simulink model "IPMSM_SVC"  (R2023a)
settings: Solver=FixedStepDiscrete  StartTime=0.0  StopTime=10.0  RelTol=1e-3
model workspace (MATLAB code in the model file):
  | cmdLim = Simulink.Parameter;
  | cmdLim.Value = 15;
  | cmdLim.Description = 'Limit for controlling the maximum surface command angle.';
  | cmdLim.Min = 0;
  | cmdLim.Max = 90;
  | cmdLim.DocUnits = 'deg';
  | 
  | dispGain = Simulink.Parameter;
  | dispGain.Value = 0.75;
  | dispGain.Description = 'Gain applied to the displacement error.';
  | dispGain.Min = 0;
  | dispGain.Max = [];
  | dispGain.DocUnits = 'deg/sec/deg';
  | 
  | dispLim = Simulink.Parameter;
  | dispLim.Value = 30;
  | dispLim.Description = 'Limit for controlling the maximum commanded angle.';
  | dispLim.Min = 0;
  | dispLim.Max = 180;
  | dispLim.DocUnits = 'deg';
  | 
  | intGain = Simulink.Parameter;
  | intGain.Value = 0.5;
  | intGain.Description = 'Gain applied to the integral error.';
  | intGain.Min = 0;
  | intGain.Max = [];
  | intGain.DocUnits = 'deg/sec/deg/sec';
  | 
  | intLim = Simulink.Parameter;
  | intLim.Value = 5;
  | intLim.Description = 'Limit for controlling the maximum commanded angle.';
  | intLim.Min = 0;
  | intLim.Max = 90;
  | intLim.DocUnits = 'deg';
  | 
  | rateGain = Simulink.Parameter;
  | rateGain.Value = 2;
  | rateGain.Description = 'Gain applied to the rate error.';
  | rateGain.Min = 0;
  | rateGain.Max = [];
  | rateGain.DocUnits = 'deg/deg/sec';
  | 
  | rateLim = Simulink.Parameter;
  | rateLim.Value = 6;
  | rateLim.Description = 'Limit for controlling the maximum commanded angle.';
  | rateLim.Min = 0;
  | rateLim.Max = 180;
  | rateLim.DocUnits = 'deg/sec';
  | 
  | hdgGain = Simulink.Parameter;
  | hdgGain.Value = 0.015;
settings Model: RequirementInfo={} %GIDa_fe9045fd_0412_4b6e_8206_617cc20e6fde  Creator=洲  LastModifiedBy=洲
settings SolverCC: AlgebraicLoopSolver=TrustRegion  AutoInsertRateTranBlk=on
settings DataIOCC: SaveOutput=off  SignalLogging=off  DSMLogging=off  SaveTime=off
settings OptimizationCC: DefaultParameterBehavior=Inlined  UseDivisionForNetSlopeComputation=on  GainParamInheritBuiltInType=on  UseFloatMulNetSlope=on  UseSpecifiedMinMax=on  InlineInvariantSignals=on  EnhancedBackFolding=on  PassReuseOutputArgsAs=Individual arguments  ZeroExternalMemoryAtStartup=off  ZeroInternalMemoryAtStartup=off  NoFixptDivByZeroProtection=on  EfficientFloat2IntCast=on  LifeSpan=1  OptimizeBlockOrder=speed  DifferentSizesBufferReuse=on  OptimizationCustomize=off  EfficientTunableParamExpr=on
settings DebuggingCC: AllowSymbolicDim=off  SFUnexpectedBacktrackingDiag=warning  SFNoUnconditionalDefaultTransitionDiag=warning  SFExecutionAtInitializationDiag=none  ArithmeticOperatorsInVariantConditions=warning
settings HardwareCC: ProdLongLongMode=on
settings SFSimCC: MATLABDynamicMemAlloc=off
settings RTWCC: Description=Embedded Coder  SystemTargetFile=ert.tlc  TemplateMakefile=ert_default_tmf  BuildConfiguration=Faster Runs  DataTypeReplacement=CDataTypesFixedWidth
settings CodeAppCC: ForceParamTrailComments=on  IgnoreCustomStorageClasses=off  OperatorAnnotations=on  SimulinkDataObjDesc=on  SFDataObjDesc=on  CustomSymbolStrGlobalVar=rt$N$M  CustomSymbolStrType=$N$M  CustomSymbolStrFcn=$N$M$F  CustomSymbolStrMacro=$N$M  InsertBlockDesc=on  EnableCustomComments=on  ReqsInCode=on
settings ERTTargetCC: TargetLangStandard=C99 (ISO)  UtilityFuncGeneration=Shared location  MultiwordLength=2048  GenerateSampleERTMain=on  IncludeMdlTerminateFcn=off  CombineSignalStateStructs=on  SuppressErrorStatus=on  SupportAbsoluteTime=off  SupportNonFinite=off  SupportComplex=off  InlinedParameterPlacement=NonHierarchical  ERTCustomFileTemplate=example_file_process.tlc  ERTFilePackagingFormat=CompactWithDataFile
settings ConfigComp: CovScope=ReferencedModels  CovSaveName=covdata_rollAP  CovMetricSettings=dcmtrwe  CovHTMLOptions=-sRT=1 -aTS=1 -bRG=1 -bTC=1 -hTR=1 -nFC=0 -scm=1 -bcm=1 -xEv=0  CovSaveCumulativeToWorkspaceVar=on  CovSaveSingleToWorkspaceVar=on  CovCumulativeVarName=covCumulativeData_rollAP  CovReportOnPause=off  CovExternalEMLEnable=off  CovSFcnEnable=off

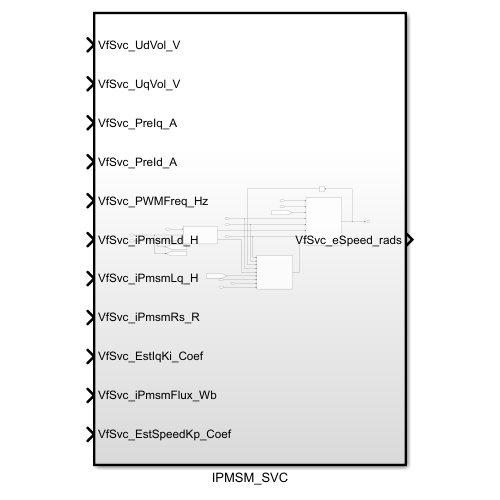
[thumbnail: Simulink's stored preview of the top-level diagram]
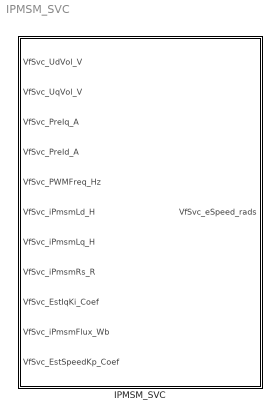
== system IPMSM_SVC ==
  IPMSM_SVC : Subsystem  TreatAsAtomicUnit=on
      settings: RTWSystemCode=Nonreusable function

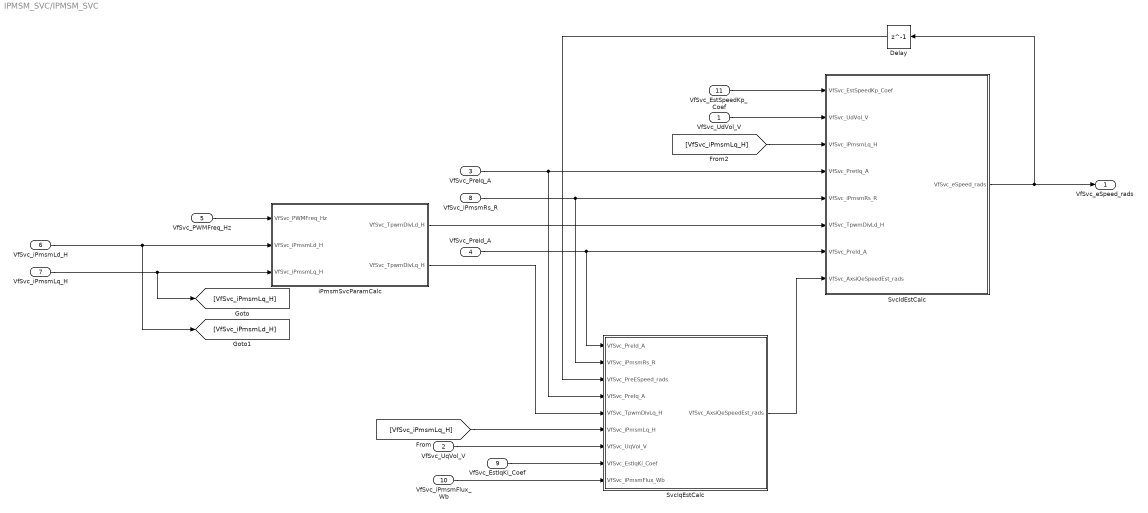
== system IPMSM_SVC/IPMSM_SVC ==
  VfSvc_UdVol_V : Inport
  VfSvc_UqVol_V : Inport  Port=2
  VfSvc_PreIq_A : Inport  Port=3
  VfSvc_PreId_A : Inport  Port=4
  VfSvc_PWMFreq_Hz : Inport  Port=5
  VfSvc_iPmsmLd_H : Inport  Port=6
  VfSvc_iPmsmLq_H : Inport  Port=7
  VfSvc_iPmsmRs_R : Inport  Port=8
  VfSvc_EstIqKi_Coef : Inport  Port=9
  VfSvc_iPmsmFlux_Wb : Inport  Port=10
  VfSvc_EstSpeedKp_Coef : Inport  Port=11
  Delay : Delay  DelayLength=1
  SvcIdEstCalc : Subsystem
  SvcIqEstCalc : Subsystem
  iPmsmSvcParamCalc : Subsystem  TreatAsAtomicUnit=on
      settings: RTWSystemCode=Nonreusable function  RTWFcnNameOpts=Use subsystem name
  VfSvc_eSpeed_rads : Outport
  wires:
  iPmsmSvcParamCalc/1(VfSvc_TpwmDivLd_H) -> SvcIdEstCalc/6(VfSvc_TpwmDivLd_H)
  SvcIqEstCalc/1(VfSvc_AxsiQeSpeedEst_rads) -> SvcIdEstCalc/8(VfSvc_AxsiQeSpeedEst_rads)
  VfSvc_iPmsmLq_H/1 -> iPmsmSvcParamCalc/3(VfSvc_iPmsmLq_H), [VfSvc_iPmsmLq_H]
  VfSvc_PreIq_A/1 -> SvcIqEstCalc/4(VfSvc_PreIq_A), SvcIdEstCalc/4(VfSvc_PretIq_A)
  VfSvc_iPmsmFlux_Wb/1 -> SvcIqEstCalc/9(VfSvc_iPmsmFlux_Wb)
  VfSvc_iPmsmRs_R/1 -> SvcIqEstCalc/2(VfSvc_iPmsmRs_R), SvcIdEstCalc/5(VfSvc_iPmsmRs_R)
  VfSvc_PWMFreq_Hz/1 -> iPmsmSvcParamCalc/1(VfSvc_PWMFreq_Hz)
  SvcIdEstCalc/1(VfSvc_eSpeed_rads) -> VfSvc_eSpeed_rads/1, Delay/1
  iPmsmSvcParamCalc/2(VfSvc_TpwmDivLq_H) -> SvcIqEstCalc/5(VfSvc_TpwmDivLq_H)
  VfSvc_PreId_A/1 -> SvcIqEstCalc/1(VfSvc_PreId_A), SvcIdEstCalc/7(VfSvc_PreId_A)
  VfSvc_iPmsmLd_H/1 -> [VfSvc_iPmsmLd_H], iPmsmSvcParamCalc/2(VfSvc_iPmsmLd_H)
  VfSvc_UdVol_V/1 -> SvcIdEstCalc/2(VfSvc_UdVol_V)
  VfSvc_UqVol_V/1 -> SvcIqEstCalc/7(VfSvc_UqVol_V)
  [VfSvc_iPmsmLq_H] -> SvcIqEstCalc/6(VfSvc_iPmsmLq_H)
  VfSvc_EstIqKi_Coef/1 -> SvcIqEstCalc/8(VfSvc_EstIqKi_Coef)
  VfSvc_EstSpeedKp_Coef/1 -> SvcIdEstCalc/1(VfSvc_EstSpeedKp_Coef)
  Delay/1 -> SvcIqEstCalc/3(VfSvc_PreESpeed_rads)
  [VfSvc_iPmsmLq_H] -> SvcIdEstCalc/3(VfSvc_iPmsmLq_H)

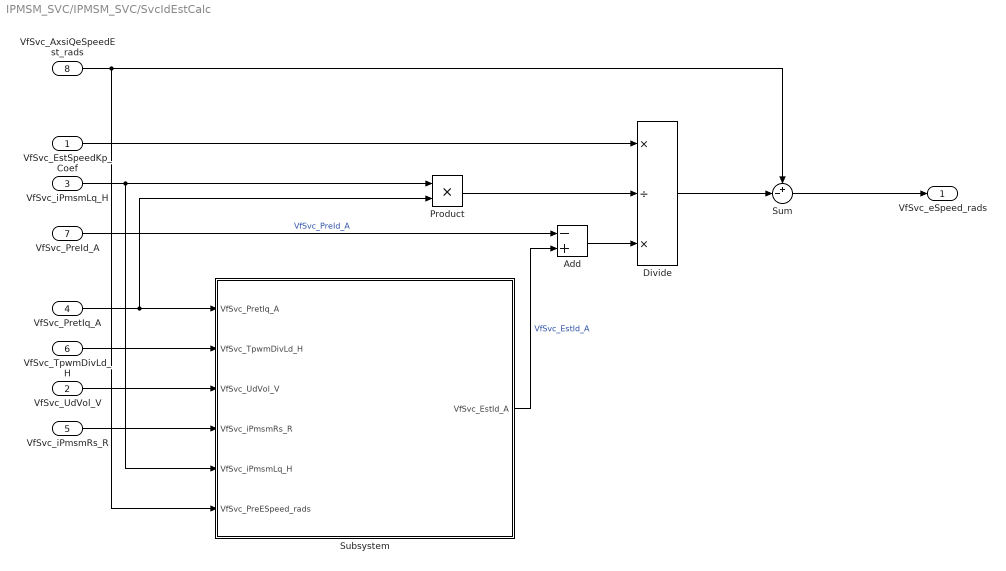
== system IPMSM_SVC/IPMSM_SVC/SvcIdEstCalc ==
  VfSvc_EstSpeedKp_Coef : Inport
  VfSvc_UdVol_V : Inport  Port=2
  VfSvc_iPmsmLq_H : Inport  Port=3
  VfSvc_PretIq_A : Inport  Port=4
  VfSvc_iPmsmRs_R : Inport  Port=5
  VfSvc_TpwmDivLd_H : Inport  Port=6
  VfSvc_PreId_A : Inport  Port=7
  VfSvc_AxsiQeSpeedEst_rads : Inport  Port=8
  Add : Sum  Inputs=-+
  Divide : Product  Inputs=*/*
  Product : Product
  Subsystem : Subsystem
  Sum : Sum  Inputs=+-|
  VfSvc_eSpeed_rads : Outport
  wires:
  VfSvc_TpwmDivLd_H/1 -> Subsystem/2(VfSvc_TpwmDivLd_H)
  VfSvc_UdVol_V/1 -> Subsystem/3(VfSvc_UdVol_V)
  VfSvc_PretIq_A/1 -> Product/2, Subsystem/1(VfSvc_PretIq_A)
  VfSvc_iPmsmRs_R/1 -> Subsystem/4(VfSvc_iPmsmRs_R)
  VfSvc_iPmsmLq_H/1 -> Subsystem/5(VfSvc_iPmsmLq_H), Product/1
  Subsystem/1(VfSvc_EstId_A) -> Add/2  "VfSvc_EstId_A"
  VfSvc_EstSpeedKp_Coef/1 -> Divide/1
  Add/1 -> Divide/3
  VfSvc_PreId_A/1 -> Add/1  "VfSvc_PreId_A"
  Divide/1 -> Sum/2
  VfSvc_AxsiQeSpeedEst_rads/1 -> Sum/1, Subsystem/6(VfSvc_PreESpeed_rads)
  Sum/1 -> VfSvc_eSpeed_rads/1
  Product/1 -> Divide/2

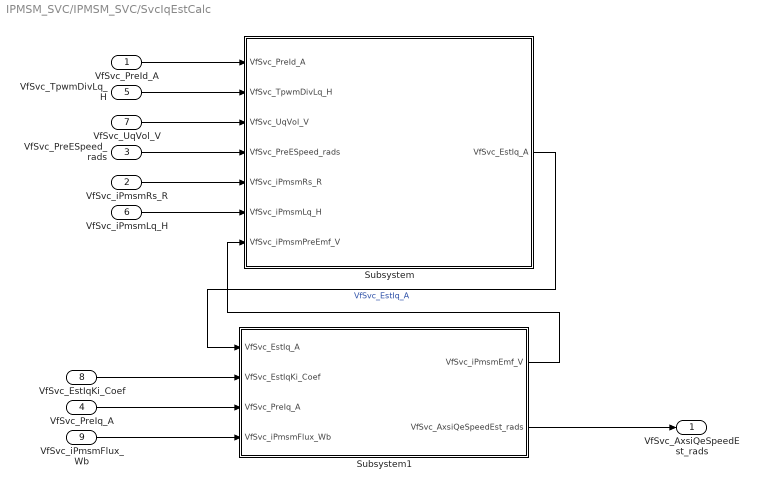
== system IPMSM_SVC/IPMSM_SVC/SvcIqEstCalc ==
  VfSvc_PreId_A : Inport
  VfSvc_iPmsmRs_R : Inport  Port=2
  VfSvc_PreESpeed_rads : Inport  Port=3
  VfSvc_PreIq_A : Inport  Port=4
  VfSvc_TpwmDivLq_H : Inport  Port=5
  VfSvc_iPmsmLq_H : Inport  Port=6
  VfSvc_UqVol_V : Inport  Port=7
  VfSvc_EstIqKi_Coef : Inport  Port=8
  VfSvc_iPmsmFlux_Wb : Inport  Port=9
  Subsystem : Subsystem
  Subsystem1 : Subsystem
  VfSvc_AxsiQeSpeedEst_rads : Outport
  wires:
  VfSvc_PreId_A/1 -> Subsystem/1(VfSvc_PreId_A)
  VfSvc_TpwmDivLq_H/1 -> Subsystem/2(VfSvc_TpwmDivLq_H)
  VfSvc_UqVol_V/1 -> Subsystem/3(VfSvc_UqVol_V)
  VfSvc_PreESpeed_rads/1 -> Subsystem/4(VfSvc_PreESpeed_rads)
  VfSvc_iPmsmRs_R/1 -> Subsystem/5(VfSvc_iPmsmRs_R)
  VfSvc_iPmsmLq_H/1 -> Subsystem/6(VfSvc_iPmsmLq_H)
  Subsystem/1(VfSvc_EstIq_A) -> Subsystem1/1(VfSvc_EstIq_A)  "VfSvc_EstIq_A"
  VfSvc_EstIqKi_Coef/1 -> Subsystem1/2(VfSvc_EstIqKi_Coef)
  VfSvc_iPmsmFlux_Wb/1 -> Subsystem1/4(VfSvc_iPmsmFlux_Wb)
  VfSvc_PreIq_A/1 -> Subsystem1/3(VfSvc_PreIq_A)
  Subsystem1/2(VfSvc_AxsiQeSpeedEst_rads) -> VfSvc_AxsiQeSpeedEst_rads/1
  Subsystem1/1(VfSvc_iPmsmEmf_V) -> Subsystem/7(VfSvc_iPmsmPreEmf_V)

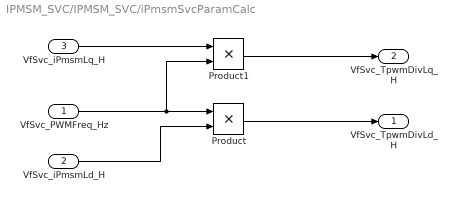
== system IPMSM_SVC/IPMSM_SVC/iPmsmSvcParamCalc ==
  VfSvc_PWMFreq_Hz : Inport
  VfSvc_iPmsmLd_H : Inport  Port=2
  VfSvc_iPmsmLq_H : Inport  Port=3
  Product : Product
  Product1 : Product
  VfSvc_TpwmDivLd_H : Outport
  VfSvc_TpwmDivLq_H : Outport  Port=2
  wires:
  VfSvc_iPmsmLq_H/1 -> Product1/1
  Product1/1 -> VfSvc_TpwmDivLq_H/1
  VfSvc_PWMFreq_Hz/1 -> Product1/2, Product/1
  Product/1 -> VfSvc_TpwmDivLd_H/1
  VfSvc_iPmsmLd_H/1 -> Product/2

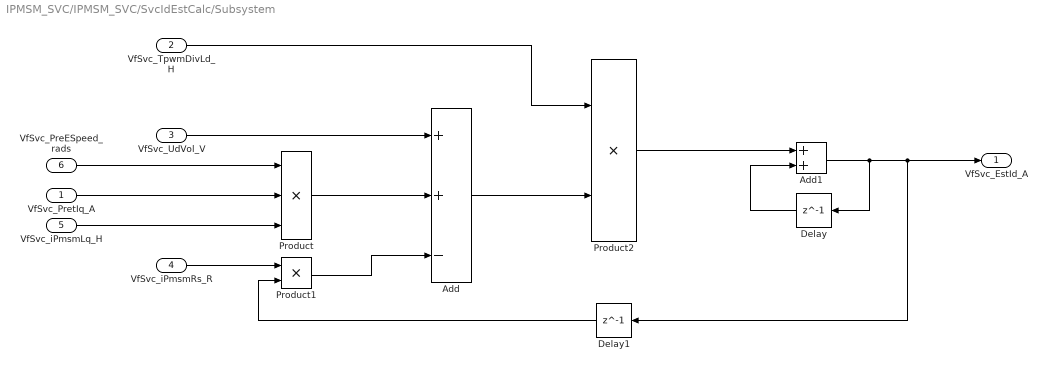
== system IPMSM_SVC/IPMSM_SVC/SvcIdEstCalc/Subsystem ==
  VfSvc_PretIq_A : Inport
  VfSvc_TpwmDivLd_H : Inport  Port=2
  VfSvc_UdVol_V : Inport  Port=3
  VfSvc_iPmsmRs_R : Inport  Port=4
  VfSvc_iPmsmLq_H : Inport  Port=5
  VfSvc_PreESpeed_rads : Inport  Port=6
  Add : Sum  Inputs=++-
  Add1 : Sum
  Delay : Delay  DelayLength=1
  Delay1 : Delay  DelayLength=1
  Product : Product  Inputs=3
  Product1 : Product
  Product2 : Product
  VfSvc_EstId_A : Outport
  wires:
  VfSvc_UdVol_V/1 -> Add/1
  VfSvc_PreESpeed_rads/1 -> Product/1
  VfSvc_TpwmDivLd_H/1 -> Product2/1
  VfSvc_PretIq_A/1 -> Product/2
  VfSvc_iPmsmRs_R/1 -> Product1/1
  Add1/1 -> Delay/1, VfSvc_EstId_A/1, Delay1/1
  Product/1 -> Add/2
  Product2/1 -> Add1/1
  Product1/1 -> Add/3
  Add/1 -> Product2/2
  Delay/1 -> Add1/2
  VfSvc_iPmsmLq_H/1 -> Product/3
  Delay1/1 -> Product1/2

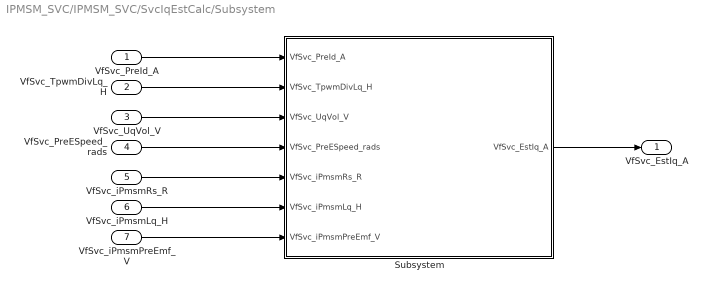
== system IPMSM_SVC/IPMSM_SVC/SvcIqEstCalc/Subsystem ==
  VfSvc_PreId_A : Inport
  VfSvc_TpwmDivLq_H : Inport  Port=2
  VfSvc_UqVol_V : Inport  Port=3
  VfSvc_PreESpeed_rads : Inport  Port=4
  VfSvc_iPmsmRs_R : Inport  Port=5
  VfSvc_iPmsmLq_H : Inport  Port=6
  VfSvc_iPmsmPreEmf_V : Inport  Port=7
  Subsystem : Subsystem
  VfSvc_EstIq_A : Outport
  wires:
  VfSvc_PreId_A/1 -> Subsystem/1(VfSvc_PreId_A)
  VfSvc_TpwmDivLq_H/1 -> Subsystem/2(VfSvc_TpwmDivLq_H)
  VfSvc_UqVol_V/1 -> Subsystem/3(VfSvc_UqVol_V)
  VfSvc_PreESpeed_rads/1 -> Subsystem/4(VfSvc_PreESpeed_rads)
  VfSvc_iPmsmRs_R/1 -> Subsystem/5(VfSvc_iPmsmRs_R)
  VfSvc_iPmsmLq_H/1 -> Subsystem/6(VfSvc_iPmsmLq_H)
  VfSvc_iPmsmPreEmf_V/1 -> Subsystem/7(VfSvc_iPmsmPreEmf_V)
  Subsystem/1(VfSvc_EstIq_A) -> VfSvc_EstIq_A/1

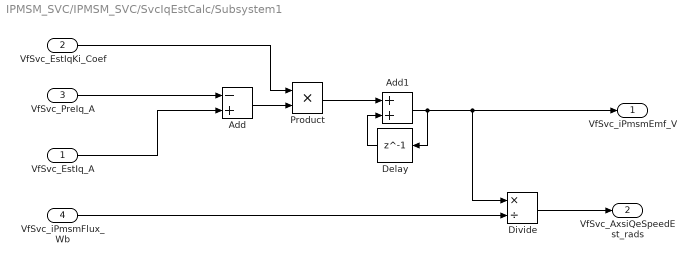
== system IPMSM_SVC/IPMSM_SVC/SvcIqEstCalc/Subsystem1 ==
  VfSvc_EstIq_A : Inport
  VfSvc_EstIqKi_Coef : Inport  Port=2
  VfSvc_PreIq_A : Inport  Port=3
  VfSvc_iPmsmFlux_Wb : Inport  Port=4
  Add : Sum  Inputs=-+
  Add1 : Sum
  Delay : Delay  DelayLength=1
  Divide : Product  Inputs=*/
  Product : Product
  VfSvc_iPmsmEmf_V : Outport
  VfSvc_AxsiQeSpeedEst_rads : Outport  Port=2
  wires:
  Product/1 -> Add1/1
  VfSvc_EstIqKi_Coef/1 -> Product/1
  VfSvc_PreIq_A/1 -> Add/1
  Add1/1 -> Divide/1, VfSvc_iPmsmEmf_V/1, Delay/1
  Add/1 -> Product/2
  Delay/1 -> Add1/2
  VfSvc_EstIq_A/1 -> Add/2
  VfSvc_iPmsmFlux_Wb/1 -> Divide/2
  Divide/1 -> VfSvc_AxsiQeSpeedEst_rads/1

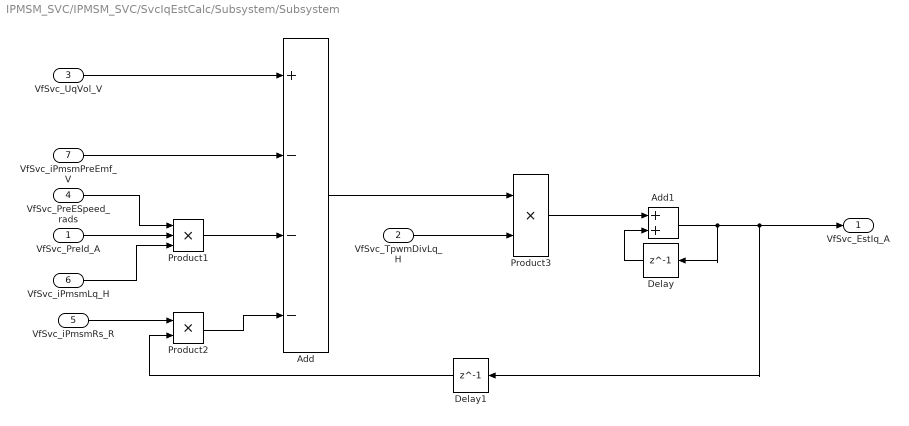
== system IPMSM_SVC/IPMSM_SVC/SvcIqEstCalc/Subsystem/Subsystem ==
  VfSvc_PreId_A : Inport
  VfSvc_TpwmDivLq_H : Inport  Port=2
  VfSvc_UqVol_V : Inport  Port=3
  VfSvc_PreESpeed_rads : Inport  Port=4
  VfSvc_iPmsmRs_R : Inport  Port=5
  VfSvc_iPmsmLq_H : Inport  Port=6
  VfSvc_iPmsmPreEmf_V : Inport  Port=7
  Add : Sum  Inputs=+---
  Add1 : Sum
  Delay : Delay  DelayLength=1
  Delay1 : Delay  DelayLength=1
  Product1 : Product  Inputs=3
  Product2 : Product
  Product3 : Product
  VfSvc_EstIq_A : Outport
  wires:
  VfSvc_iPmsmRs_R/1 -> Product2/1
  Add1/1 -> Delay/1, VfSvc_EstIq_A/1, Delay1/1
  Add/1 -> Product3/1
  VfSvc_iPmsmLq_H/1 -> Product1/3
  VfSvc_iPmsmPreEmf_V/1 -> Add/2
  Delay/1 -> Add1/2
  VfSvc_TpwmDivLq_H/1 -> Product3/2
  VfSvc_UqVol_V/1 -> Add/1
  Product3/1 -> Add1/1
  Product1/1 -> Add/3
  VfSvc_PreId_A/1 -> Product1/2
  VfSvc_PreESpeed_rads/1 -> Product1/1
  Product2/1 -> Add/4
  Delay1/1 -> Product2/2
